simulink model "psbflowsolv"  (Simulink 6.0)
settings: Solver=FixedStepDiscrete  SolverMode=SingleTasking  StartTime=0.0  StopTime=1  FixedStep=0.5  RelTol=1e-3  AbsTol=1e-2
undefined symbols (not defined in the file or in its folder): imag_current_guess, imag_Van_init, Kii, Kir, Pmec, Pref, Qref, R1, r2, real_current_guess, real_Van_init, slip_guess, t_start_current_mot, U, Uref, X1, x2
settings Model: Creator=patrice  LastModifiedBy=batserve  ExtModeTrigMode=oneshot  ExtModeArmWhenConnect=off  ExtModeAutoUpdateStatusClock=off
settings DataIOCC: LimitDataPoints=off  SignalLoggingName=sigsOut
settings OptimizationCC: BooleanDataType=off
settings DebuggingCC: AlgebraicLoopMsg=none  SolverPrmCheckMsg=none  UnconnectedInputMsg=none  UnconnectedOutputMsg=none
settings HardwareCC: TargetUnknown=on
settings RTWCC: TemplateMakefile=grt_unix.tmf

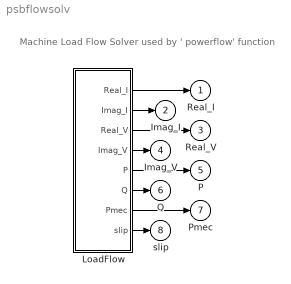
== system psbflowsolv ==
  note: Machine Load Flow Solver
      |  used by ' powerflow' function
  LoadFlow : Subsystem
  Real_I : Outport  InitialOutput=0
  Imag_I : Outport  Port=2  InitialOutput=0
  Real_V : Outport  Port=3  InitialOutput=0
  Imag_V : Outport  Port=4  InitialOutput=0
  P : Outport  Port=5  InitialOutput=0
  Q : Outport  Port=6  InitialOutput=0
  Pmec : Outport  Port=7  InitialOutput=0
  slip : Outport  Port=8  InitialOutput=0
  wires:
  LoadFlow/1(Real_I) -> Real_I/1
  LoadFlow/3(Real_V) -> Real_V/1
  LoadFlow/5(P) -> P/1
  LoadFlow/6(Q) -> Q/1
  LoadFlow/7(Pmec) -> Pmec/1
  LoadFlow/8(slip) -> slip/1
  LoadFlow/4(Imag_V) -> Imag_V/1
  LoadFlow/2(Imag_I) -> Imag_I/1

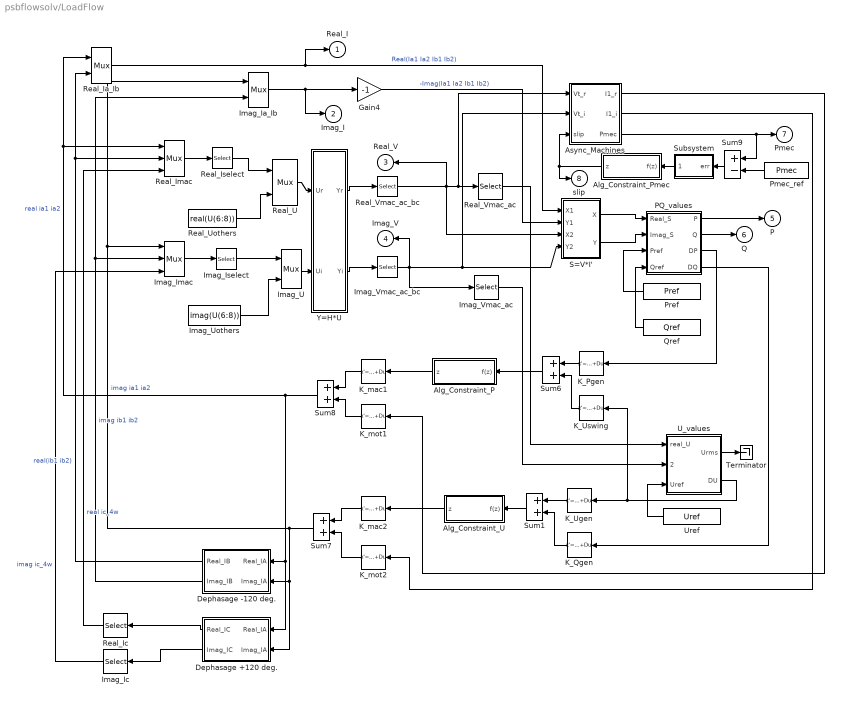
== system psbflowsolv/LoadFlow ==
  Alg_Constraint_P : Subsystem  Orientation=left  mask(Algebraic Constraint){z0=real_current_guess}
      mask prompts: z0 "Initial guess:"
      mask help: Constrains input signal f(z) to zero and outputs an algebraic state z. This block outputs the value necessary to produce a zero at the input. The output must affect the input through some feedback path. Provide an initial guess of the output to improve algebraic loop solver efficiency.
      mask Help:
      | This block outputs the value necessary to produce a zero at the input. The output must affect the input through some feedback path. This allows you to specify algebraic equations for index 1 differential/algebraic systems (DAE's).
      | 
      | By default, the initial guess is zero.  You can improve the efficiency of the algebraic loop solver by providing an initial guess that is close to the solution value.
      mask Display: disp('Solve\nf(z) = 0')
  Alg_Constraint_Pmec : Subsystem  Orientation=left  mask(Algebraic Constraint){z0=slip_guess}
      mask prompts: z0 "Initial guess:"
      mask help: Constrains input signal f(z) to zero and outputs an algebraic state z. This block outputs the value necessary to produce a zero at the input. The output must affect the input through some feedback path. Provide an initial guess of the output to improve algebraic loop solver efficiency.
      mask Help:
      | This block outputs the value necessary to produce a zero at the input. The output must affect the input through some feedback path. This allows you to specify algebraic equations for index 1 differential/algebraic systems (DAE's).
      | 
      | By default, the initial guess is zero.  You can improve the efficiency of the algebraic loop solver by providing an initial guess that is close to the solution value.
      mask Display: disp('Solve\nf(z) = 0')
  Alg_Constraint_U : Subsystem  Orientation=left  mask(Algebraic Constraint){z0=imag_current_guess}
      mask prompts: z0 "Initial guess:"
      mask help: Constrains input signal f(z) to zero and outputs an algebraic state z. This block outputs the value necessary to produce a zero at the input. The output must affect the input through some feedback path. Provide an initial guess of the output to improve algebraic loop solver efficiency.
      mask Help:
      | This block outputs the value necessary to produce a zero at the input. The output must affect the input through some feedback path. This allows you to specify algebraic equations for index 1 differential/algebraic systems (DAE's).
      | 
      | By default, the initial guess is zero.  You can improve the efficiency of the algebraic loop solver by providing an initial guess that is close to the solution value.
      mask Display: disp('Solve\nf(z) = 0')
  Async_Machines : Subsystem
  Dephasage +120 deg. : Subsystem  Orientation=left
  Dephasage -120 deg. : Subsystem  Orientation=left
  Gain4 : Gain  Gain=-1  SaturateOnIntegerOverflow=on
  Imag_Ia_Ib : Mux  Inputs=[2 2]
  Imag_Ic : Selector  Orientation=left  Elements=[1]  InputPortWidth=2
  Imag_Imac : Mux  Inputs=[2 2 1]
  Imag_Iselect : Selector  Elements=[1:5]  InputPortWidth=5
  Imag_U : Mux  Inputs=[5 3]
  Imag_Uothers : Constant  Value=imag(U(6:8))
  Imag_Vmac_ac : Selector  Elements=1:2  InputPortWidth=4
  Imag_Vmac_ac_bc : Selector  Elements=1:4  InputPortWidth=9
  K_Pgen : StateSpace  Orientation=left  A=[]  B=[]  C=[]  D=K  mask(Matrix Gain){@1=[0 0;0 1]}
      mask prompts: @1 "Gain matrix:"
      mask help: Matrix Gain.
      mask init:
      | K=@1;
      mask Help: Multiplies input vector by entered matrix to produce output vector (y=Au).
      mask Display: disp('K')
  K_Qgen : StateSpace  Orientation=left  A=[]  B=[]  C=[]  D=K  mask(Matrix Gain){@1=[0 0;0 1]}
      mask prompts: @1 "Gain matrix:"
      mask help: Matrix Gain.
      mask init:
      | K=@1;
      mask Help: Multiplies input vector by entered matrix to produce output vector (y=Au).
      mask Display: disp('K')
  K_Ugen : StateSpace  Orientation=left  A=[]  B=[]  C=[]  D=K  mask(Matrix Gain){@1=[0 0;0 0]}
      mask prompts: @1 "Gain matrix:"
      mask help: Matrix Gain.
      mask init:
      | K=@1;
      mask Help: Multiplies input vector by entered matrix to produce output vector (y=Au).
      mask Display: disp('K')
  K_Uswing : StateSpace  Orientation=left  A=[]  B=[]  C=[]  D=K  mask(Matrix Gain){@1=[1 0;0 0]}
      mask prompts: @1 "Gain matrix:"
      mask help: Matrix Gain.
      mask init:
      | K=@1;
      mask Help: Multiplies input vector by entered matrix to produce output vector (y=Au).
      mask Display: disp('K')
  K_mac1 : StateSpace  Orientation=left  A=[]  B=[]  C=[]  D=K  mask(Matrix Gain){@1=[1 0;0 1]}
      mask prompts: @1 "Gain matrix:"
      mask help: Matrix Gain.
      mask init:
      | K=@1;
      mask Help: Multiplies input vector by entered matrix to produce output vector (y=Au).
      mask Display: disp('K')
  K_mac2 : StateSpace  Orientation=left  A=[]  B=[]  C=[]  D=K  mask(Matrix Gain){@1=[1 0;0 1]}
      mask prompts: @1 "Gain matrix:"
      mask help: Matrix Gain.
      mask init:
      | K=@1;
      mask Help: Multiplies input vector by entered matrix to produce output vector (y=Au).
      mask Display: disp('K')
  K_mot1 : StateSpace  Orientation=left  A=[]  B=[]  C=[]  D=K  mask(Matrix Gain){@1=[0 0;0 0]}
      mask prompts: @1 "Gain matrix:"
      mask help: Matrix Gain.
      mask init:
      | K=@1;
      mask Help: Multiplies input vector by entered matrix to produce output vector (y=Au).
      mask Display: disp('K')
  K_mot2 : StateSpace  Orientation=left  A=[]  B=[]  C=[]  D=K  mask(Matrix Gain){@1=[0 0;0 0]}
      mask prompts: @1 "Gain matrix:"
      mask help: Matrix Gain.
      mask init:
      | K=@1;
      mask Help: Multiplies input vector by entered matrix to produce output vector (y=Au).
      mask Display: disp('K')
  PQ_values : Subsystem
  Pmec_ref : Constant  Orientation=left  Value=Pmec
  Pref : Constant  Orientation=left  Value=Pref
  Qref : Constant  Orientation=left  Value=Qref
  Real_Ia_Ib : Mux  Inputs=[2 2]
  Real_Ic : Selector  Orientation=left  Elements=[1]  InputPortWidth=2
  Real_Imac : Mux  Inputs=[2 2 1]
  Real_Iselect : Selector  Elements=[1:5]  InputPortWidth=5
  Real_U : Mux  Inputs=[5 3]
  Real_Uothers : Constant  Value=real(U(6:8))
  Real_Vmac_ac : Selector  Elements=1:2  InputPortWidth=4
  Real_Vmac_ac_bc : Selector  Elements=1:4  InputPortWidth=9
  S=V*I' : Subsystem
      mask Display: disp('Z1.*Z2')
  Subsystem : Subsystem  Orientation=left
  Sum{1,6..8} (4 alike) : Sum  Orientation=left  SaturateOnIntegerOverflow=on  InputSameDT=on
  Sum9 : Sum  Orientation=left  Inputs=+-  SaturateOnIntegerOverflow=on  InputSameDT=on
  Terminator : Terminator
  U_values : Subsystem
  Uref : Constant  Orientation=left  Value=Uref
  Y=H*U : Subsystem
      mask Display: disp('Y=H*U')
  Real_I : Outport  InitialOutput=0
  Imag_I : Outport  Port=2  InitialOutput=0
  Real_V : Outport  Orientation=left  Port=3  InitialOutput=0
  Imag_V : Outport  Orientation=left  Port=4  InitialOutput=0
  P : Outport  Port=5  InitialOutput=0
  Q : Outport  Port=6  InitialOutput=0
  Pmec : Outport  Port=7  InitialOutput=0
  slip : Outport  Port=8  InitialOutput=0
  wires:
  Subsystem/1(Psolv) -> Alg_Constraint_Pmec/1(f(z))
  Sum9/1 -> Subsystem/1(err)
  Pmec_ref/1 -> Sum9/2
  Async_Machines/3(Pmec) -> Sum9/1, Pmec/1
  K_mot2/1 -> Sum7/2
  Real_Vmac_ac_bc/1 -> Async_Machines/1(Vt_r), Real_V/1, S=V*I'/3(X2), Real_Vmac_ac/1
  Sum8/1 -> Dephasage -120 deg./1(Real_IA), Dephasage +120 deg./1(Real_IA), Real_Imac/1, Real_Ia_Ib/1  "real ia1 ia2"
  Sum6/1 -> Alg_Constraint_P/1(f(z))
  K_Uswing/1 -> Sum6/2
  K_Pgen/1 -> Sum6/1
  Imag_Vmac_ac_bc/1 -> Async_Machines/2(Vt_i), S=V*I'/4(Y2), Imag_V/1, Imag_Vmac_ac/1
  Real_U/1 -> Y=H*U/1(Ur)
  Y=H*U/2(Yi) -> Imag_Vmac_ac_bc/1
  Y=H*U/1(Yr) -> Real_Vmac_ac_bc/1
  Imag_U/1 -> Y=H*U/2(Ui)
  Gain4/1 -> S=V*I'/2(Y1)  "-Imag(Ia1 Ia2 Ib1 Ib2)"
  U_values/2(DU) -> K_Uswing/1, K_Ugen/1
  PQ_values/2(Q) -> Q/1
  S=V*I'/2(Y) -> PQ_values/2(Imag_S)
  PQ_values/1(P) -> P/1
  Pref/1 -> PQ_values/3(Pref)
  S=V*I'/1(X) -> PQ_values/1(Real_S)
  Imag_Vmac_ac/1 -> U_values/2(imag_U)
  Real_Vmac_ac/1 -> U_values/1(real_U)
  Uref/1 -> U_values/3(Uref)
  PQ_values/3(DP) -> K_Pgen/1
  Imag_Uothers/1 -> Imag_U/2
  Real_Uothers/1 -> Real_U/2
  Alg_Constraint_U/1(z) -> K_mac2/1
  K_mac2/1 -> Sum7/1
  Async_Machines/2(I1_i) -> K_mot2/1
  Dephasage -120 deg./1("Real_IB ") -> Real_Imac/2, Real_Ia_Ib/2  "real(ib1 ib2)"
  Dephasage -120 deg./2("Imag_IB ") -> Imag_Imac/2, Imag_Ia_Ib/2  "imag ib1 ib2"
  Sum7/1 -> Dephasage -120 deg./2(Imag_IA), Dephasage +120 deg./2(Imag_IA), Imag_Imac/1, Imag_Ia_Ib/1  "imag ia1 ia2"
  Alg_Constraint_P/1(z) -> K_mac1/1
  K_mac1/1 -> Sum8/1
  Async_Machines/1(I1_r) -> K_mot1/1
  K_mot1/1 -> Sum8/2
  Alg_Constraint_Pmec/1(z) -> Async_Machines/3(slip), slip/1
  Sum1/1 -> Alg_Constraint_U/1(f(z))
  K_Ugen/1 -> Sum1/1
  K_Qgen/1 -> Sum1/2
  Qref/1 -> PQ_values/4(Qref)
  PQ_values/4(DQ) -> K_Qgen/1
  Dephasage +120 deg./1("Real_IC ") -> Real_Ic/1
  Dephasage +120 deg./2("Imag_IC ") -> Imag_Ic/1
  Real_Ic/1 -> Real_Imac/3  "real ic_4w"
  Imag_Ic/1 -> Imag_Imac/3  "imag ic_4w"
  Real_Ia_Ib/1 -> S=V*I'/1(X1), Real_I/1  "Real(Ia1 Ia2 Ib1 Ib2)"
  Imag_Ia_Ib/1 -> Gain4/1, Imag_I/1
  U_values/1(Urms) -> Terminator/1
  Real_Imac/1 -> Real_Iselect/1
  Real_Iselect/1 -> Real_U/1
  Imag_Imac/1 -> Imag_Iselect/1
  Imag_Iselect/1 -> Imag_U/1

== system psbflowsolv/LoadFlow/Alg_Constraint_P ==
  f(z) : Inport  Port=1  LatchInput=off
  Initial Guess : InitialCondition  Value=z0
  Sum : Sum  SaturateOnIntegerOverflow=on  InputSameDT=on
  z : Outport  InitialOutput=0
  wires:
  Sum/1 -> Initial Guess/1
  Initial Guess/1 -> Sum/2, z/1
  f(z)/1 -> Sum/1

== system psbflowsolv/LoadFlow/Alg_Constraint_Pmec ==
  f(z) : Inport  Port=1  LatchInput=off
  Initial Guess : InitialCondition  Value=z0
  Sum : Sum  SaturateOnIntegerOverflow=on  InputSameDT=on
  z : Outport  InitialOutput=0
  wires:
  f(z)/1 -> Sum/1
  Initial Guess/1 -> z/1, Sum/2
  Sum/1 -> Initial Guess/1

== system psbflowsolv/LoadFlow/Alg_Constraint_U ==
  f(z) : Inport  Port=1  LatchInput=off
  Initial Guess : InitialCondition  Value=z0
  Sum : Sum  SaturateOnIntegerOverflow=on  InputSameDT=on
  z : Outport  InitialOutput=0
  wires:
  Sum/1 -> Initial Guess/1
  Initial Guess/1 -> Sum/2, z/1
  f(z)/1 -> Sum/1

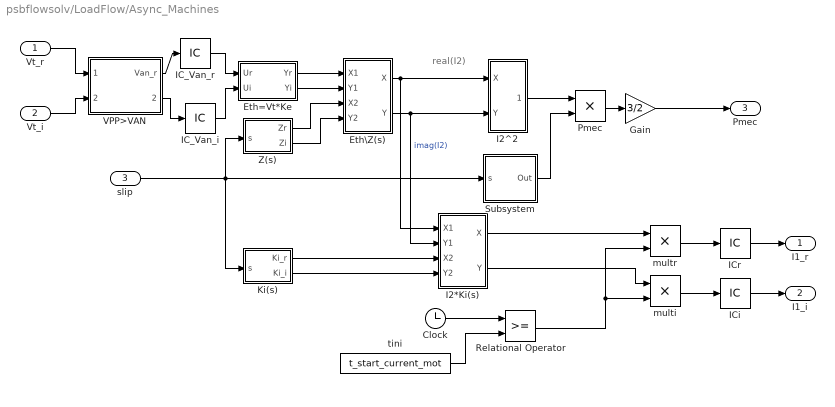
== system psbflowsolv/LoadFlow/Async_Machines ==
  note: real(I2)
  Vt_r : Inport  Port=1  LatchInput=off
  Vt_i : Inport  Port=2  LatchInput=off
  slip : Inport  Port=3  LatchInput=off
  Clock : Clock
      settings: Decimation=10
  Eth=Vt*Ke : Subsystem
      mask Display: disp('Y=H*U')
  Eth\Z(s) : Subsystem
      mask Display: disp('Z1./Z2')
  Gain : Gain  Gain=3/2  SaturateOnIntegerOverflow=on
  I2*Ki(s) : Subsystem
      mask Display: disp('Z1.*Z2')
  I2^2 : Subsystem
  IC_Van_i : InitialCondition  Value=imag_Van_init
  IC_Van_r : InitialCondition  Value=real_Van_init
  ICi : InitialCondition  Value=0
  ICr : InitialCondition  Value=0
  Ki(s) : Subsystem
  "Pmec " : Product  SaturateOnIntegerOverflow=on  InputSameDT=on
  Relational Operator : RelationalOperator  InputSameDT=on
  Subsystem : Subsystem
      mask Display: disp('r2(1-s)/s')
  VPP>VAN : Subsystem
  Z(s) : Subsystem
  "multi " : Product  SaturateOnIntegerOverflow=on  InputSameDT=on
  multr : Product  SaturateOnIntegerOverflow=on  InputSameDT=on
  tini : Constant  Value=t_start_current_mot
  I1_r : Outport  InitialOutput=0
  I1_i : Outport  Port=2  InitialOutput=0
  Pmec : Outport  Port=3  InitialOutput=0
  wires:
  IC_Van_i/1 -> Eth=Vt*Ke/2(Ui)
  VPP>VAN/2(Van_r1) -> IC_Van_i/1
  VPP>VAN/1(Van_r) -> IC_Van_r/1
  IC_Van_r/1 -> Eth=Vt*Ke/1(Ur)
  Relational Operator/1 -> multr/2, "multi "/2
  I2*Ki(s)/2(Y) -> "multi "/1
  I2*Ki(s)/1(X) -> multr/1
  tini/1 -> Relational Operator/2
  Clock/1 -> Relational Operator/1
  Eth\Z(s)/2(Y) -> I2*Ki(s)/2(Y1), I2^2/2(Y)  "imag(I2)"
  Eth\Z(s)/1(X) -> I2*Ki(s)/1(X1), I2^2/1(X)
  Ki(s)/2(Ki_i) -> I2*Ki(s)/4(Y2)
  Ki(s)/1(Ki_r) -> I2*Ki(s)/3(X2)
  Gain/1 -> Pmec/1
  "Pmec "/1 -> Gain/1
  Z(s)/1(Zr) -> Eth\Z(s)/3(X2)
  Z(s)/2(Zi) -> Eth\Z(s)/4(Y2)
  slip/1 -> Ki(s)/1(s), Subsystem/1(s), Z(s)/1(s)
  Subsystem/1(Out) -> "Pmec "/2
  Eth=Vt*Ke/1(Yr) -> Eth\Z(s)/1(X1)
  Eth=Vt*Ke/2(Yi) -> Eth\Z(s)/2(Y1)
  I2^2/1(|Z|^2) -> "Pmec "/1
  multr/1 -> ICr/1
  ICr/1 -> I1_r/1
  "multi "/1 -> ICi/1
  ICi/1 -> I1_i/1
  Vt_r/1 -> VPP>VAN/1(Vac_bc_r)
  Vt_i/1 -> VPP>VAN/2(Vac_bc_i)

== system psbflowsolv/LoadFlow/Dephasage +120 deg. ==
  Real_IA : Inport  Orientation=left  Port=1  LatchInput=off
  Imag_IA : Inport  Orientation=left  Port=2  LatchInput=off
  Mult. complex : Subsystem  Orientation=left
      mask Display: disp('Z1.*Z2')
  imagl(a) : Constant  Orientation=left  Value=sqrt(3)/2
  real(a) : Constant  Orientation=left  Value=-0.5
  "Real_IC " : Outport  Orientation=left  InitialOutput=0
  "Imag_IC " : Outport  Orientation=left  Port=2  InitialOutput=0
  wires:
  Mult. complex/2(Y) -> "Imag_IC "/1
  Mult. complex/1(X) -> "Real_IC "/1
  Real_IA/1 -> Mult. complex/1(X1)
  Imag_IA/1 -> Mult. complex/2(Y1)
  real(a)/1 -> Mult. complex/3(X2)
  imagl(a)/1 -> Mult. complex/4(Y2)

== system psbflowsolv/LoadFlow/Dephasage -120 deg. ==
  Real_IA : Inport  Orientation=left  Port=1  LatchInput=off
  Imag_IA : Inport  Orientation=left  Port=2  LatchInput=off
  Mult. complex : Subsystem  Orientation=left
      mask Display: disp('Z1.*Z2')
  imagl(a^2) : Constant  Orientation=left  Value=-sqrt(3)/2
  real(a^2) : Constant  Orientation=left  Value=-0.5
  "Real_IB " : Outport  Orientation=left  InitialOutput=0
  "Imag_IB " : Outport  Orientation=left  Port=2  InitialOutput=0
  wires:
  imagl(a^2)/1 -> Mult. complex/4(Y2)
  real(a^2)/1 -> Mult. complex/3(X2)
  Imag_IA/1 -> Mult. complex/2(Y1)
  Real_IA/1 -> Mult. complex/1(X1)
  Mult. complex/1(X) -> "Real_IB "/1
  Mult. complex/2(Y) -> "Imag_IB "/1

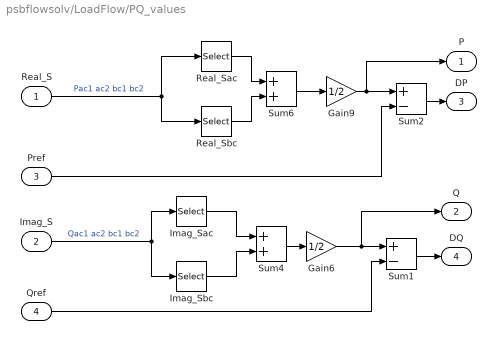
== system psbflowsolv/LoadFlow/PQ_values ==
  Real_S : Inport  Port=1  LatchInput=off
  Imag_S : Inport  Port=2  LatchInput=off
  Pref : Inport  Port=3  LatchInput=off
  Qref : Inport  Port=4  LatchInput=off
  Gain6 : Gain  Gain=1/2  SaturateOnIntegerOverflow=on
  Gain9 : Gain  Gain=1/2  SaturateOnIntegerOverflow=on
  Imag_Sac : Selector  Elements=1:2  InputPortWidth=4
  Imag_Sbc : Selector  Elements=3:4  InputPortWidth=4
  Real_Sac : Selector  Elements=1:2  InputPortWidth=4
  Real_Sbc : Selector  Elements=3:4  InputPortWidth=4
  Sum1 : Sum  Inputs=+-  SaturateOnIntegerOverflow=on  InputSameDT=on
  Sum2 : Sum  Inputs=+-  SaturateOnIntegerOverflow=on  InputSameDT=on
  Sum4 : Sum  SaturateOnIntegerOverflow=on  InputSameDT=on
  Sum6 : Sum  SaturateOnIntegerOverflow=on  InputSameDT=on
  P : Outport  InitialOutput=0
  Q : Outport  Port=2  InitialOutput=0
  DP : Outport  Port=3  InitialOutput=0
  DQ : Outport  Port=4  InitialOutput=0
  wires:
  Imag_S/1 -> Imag_Sac/1, Imag_Sbc/1  "Qac1 ac2 bc1 bc2"
  Sum4/1 -> Gain6/1
  Imag_Sbc/1 -> Sum4/2
  Imag_Sac/1 -> Sum4/1
  Gain9/1 -> P/1, Sum2/1
  Sum2/1 -> DP/1
  Pref/1 -> Sum2/2
  Sum6/1 -> Gain9/1
  Real_Sbc/1 -> Sum6/2
  Real_Sac/1 -> Sum6/1
  Real_S/1 -> Real_Sbc/1, Real_Sac/1  "Pac1 ac2 bc1 bc2"
  Gain6/1 -> Sum1/1, Q/1
  Sum1/1 -> DQ/1
  Qref/1 -> Sum1/2

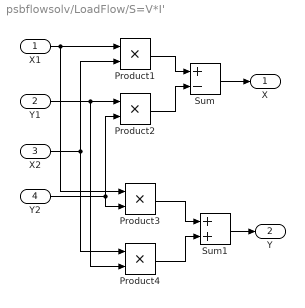
== system psbflowsolv/LoadFlow/S=V*I' ==
  X1 : Inport  Port=1  LatchInput=off
  Y1 : Inport  Port=2  LatchInput=off
  X2 : Inport  Port=3  LatchInput=off
  Y2 : Inport  Port=4  LatchInput=off
  Product{1..4} (4 alike) : Product  SaturateOnIntegerOverflow=on  InputSameDT=on
  Sum : Sum  Inputs=+-  SaturateOnIntegerOverflow=on  InputSameDT=on
  Sum1 : Sum  SaturateOnIntegerOverflow=on  InputSameDT=on
  X : Outport  InitialOutput=0
  Y : Outport  Port=2  InitialOutput=0
  wires:
  Y1/1 -> Product4/2, Product2/1
  X2/1 -> Product4/1, Product1/2
  Y2/1 -> Product3/2, Product2/2
  X1/1 -> Product3/1, Product1/1
  Product3/1 -> Sum1/1
  Product4/1 -> Sum1/2
  Sum1/1 -> Y/1
  Product2/1 -> Sum/2
  Product1/1 -> Sum/1
  Sum/1 -> X/1

== system psbflowsolv/LoadFlow/Subsystem ==
  err : Inport  Port=1  LatchInput=off
  Clock : Clock
      settings: Decimation=10
  Relational Operator : RelationalOperator  InputSameDT=on
  "multi " : Product  SaturateOnIntegerOverflow=on  InputSameDT=on
  tini : Constant  Value=t_start_current_mot
  Psolv : Outport  InitialOutput=0
  wires:
  "multi "/1 -> Psolv/1
  err/1 -> "multi "/1
  tini/1 -> Relational Operator/2
  Clock/1 -> Relational Operator/1
  Relational Operator/1 -> "multi "/2

== system psbflowsolv/LoadFlow/U_values ==
  real_U : Inport  Port=1  LatchInput=off
  imag_U : Inport  Port=2  LatchInput=off
  Uref : Inport  Port=3  LatchInput=off
  Cartesian to Polar2 : Subsystem
      mask Type: Cart2Polar
      mask Description:
      | Transformation from cartesian to polar coordinates.
      | [x, y] -> [r, theta]
      | 
      | r = sqrt(x^2 + y^2);
      | theta = atan(y/x);
      mask Help: Unmask this block for more help.
      mask Display: plot(0,0,100,100,[24,20,15,20,20],[85,95,85,95,20],[80,20,95,85,95,85],[70,20,20,15,20,24],[56,56,55,52,50,46],[20,26,31,35,38,42])
  Sum5 : Sum  Inputs=+-  SaturateOnIntegerOverflow=on  InputSameDT=on
  Vrms : Gain  Gain=1/sqrt(2)  SaturateOnIntegerOverflow=on
  Urms : Outport  InitialOutput=0
  DU : Outport  Port=2  InitialOutput=0
  wires:
  Vrms/1 -> Sum5/1, Urms/1
  real_U/1 -> Cartesian to Polar2/1(x)
  imag_U/1 -> Cartesian to Polar2/2(y)
  Cartesian to Polar2/1(r) -> Vrms/1
  Sum5/1 -> DU/1
  Uref/1 -> Sum5/2

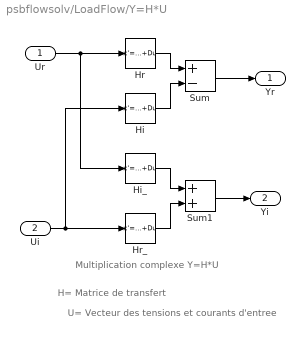
== system psbflowsolv/LoadFlow/Y=H*U ==
  note: Multiplication complexe Y=H*U
  note: H= Matrice de transfert
  note: U= Vecteur des tensions et courants d'entree
  Ur : Inport  Port=1  LatchInput=off
  Ui : Inport  Port=2  LatchInput=off
  Hi : StateSpace  A=[]  B=[]  C=[]  D=K  mask(Matrix Gain){@1=imag(H)}
      mask prompts: @1 "Gain matrix:"
      mask help: Matrix Gain.
      mask init:
      | K=@1;
      mask Help: Multiplies input vector by entered matrix to produce output vector (y=Au).
      mask Display: disp('K')
  Hi_ : StateSpace  A=[]  B=[]  C=[]  D=K  mask(Matrix Gain){@1=imag(H)}
      mask prompts: @1 "Gain matrix:"
      mask help: Matrix Gain.
      mask init:
      | K=@1;
      mask Help: Multiplies input vector by entered matrix to produce output vector (y=Au).
      mask Display: disp('K')
  Hr : StateSpace  A=[]  B=[]  C=[]  D=K  mask(Matrix Gain){@1=real(H)}
      mask prompts: @1 "Gain matrix:"
      mask help: Matrix Gain.
      mask init:
      | K=@1;
      mask Help: Multiplies input vector by entered matrix to produce output vector (y=Au).
      mask Display: disp('K')
  Hr_ : StateSpace  A=[]  B=[]  C=[]  D=K  mask(Matrix Gain){@1=real(H)}
      mask prompts: @1 "Gain matrix:"
      mask help: Matrix Gain.
      mask init:
      | K=@1;
      mask Help: Multiplies input vector by entered matrix to produce output vector (y=Au).
      mask Display: disp('K')
  Sum : Sum  Inputs=+-  SaturateOnIntegerOverflow=on  InputSameDT=on
  Sum1 : Sum  SaturateOnIntegerOverflow=on  InputSameDT=on
  Yr : Outport  InitialOutput=0
  Yi : Outport  Port=2  InitialOutput=0
  wires:
  Hr/1 -> Sum/1
  Hi/1 -> Sum/2
  Sum/1 -> Yr/1
  Ur/1 -> Hr/1, Hi_/1
  Ui/1 -> Hi/1, Hr_/1
  Hi_/1 -> Sum1/1
  Hr_/1 -> Sum1/2
  Sum1/1 -> Yi/1

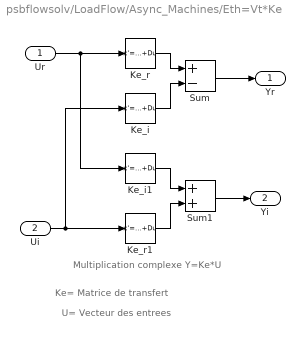
== system psbflowsolv/LoadFlow/Async_Machines/Eth=Vt*Ke ==
  note: Multiplication complexe Y=Ke*U
  note: Ke= Matrice de transfert
  note: U= Vecteur des entrees
  Ur : Inport  Port=1  LatchInput=off
  Ui : Inport  Port=2  LatchInput=off
  Ke_i : StateSpace  A=[]  B=[]  C=[]  D=K  mask(Matrix Gain){@1=imag(Ke)}
      mask prompts: @1 "Gain matrix:"
      mask help: Matrix Gain.
      mask init:
      | K=@1;
      mask Help: Multiplies input vector by entered matrix to produce output vector (y=Au).
      mask Display: disp('K')
  Ke_i1 : StateSpace  A=[]  B=[]  C=[]  D=K  mask(Matrix Gain){@1=imag(Ke)}
      mask prompts: @1 "Gain matrix:"
      mask help: Matrix Gain.
      mask init:
      | K=@1;
      mask Help: Multiplies input vector by entered matrix to produce output vector (y=Au).
      mask Display: disp('K')
  Ke_r : StateSpace  A=[]  B=[]  C=[]  D=K  mask(Matrix Gain){@1=real(Ke)}
      mask prompts: @1 "Gain matrix:"
      mask help: Matrix Gain.
      mask init:
      | K=@1;
      mask Help: Multiplies input vector by entered matrix to produce output vector (y=Au).
      mask Display: disp('K')
  Ke_r1 : StateSpace  A=[]  B=[]  C=[]  D=K  mask(Matrix Gain){@1=real(Ke)}
      mask prompts: @1 "Gain matrix:"
      mask help: Matrix Gain.
      mask init:
      | K=@1;
      mask Help: Multiplies input vector by entered matrix to produce output vector (y=Au).
      mask Display: disp('K')
  Sum : Sum  Inputs=+-  SaturateOnIntegerOverflow=on  InputSameDT=on
  Sum1 : Sum  SaturateOnIntegerOverflow=on  InputSameDT=on
  Yr : Outport  InitialOutput=0
  Yi : Outport  Port=2  InitialOutput=0
  wires:
  Ke_r/1 -> Sum/1
  Ke_i/1 -> Sum/2
  Sum/1 -> Yr/1
  Ui/1 -> Ke_i/1, Ke_r1/1
  Ke_i1/1 -> Sum1/1
  Ke_r1/1 -> Sum1/2
  Sum1/1 -> Yi/1
  Ur/1 -> Ke_r/1, Ke_i1/1

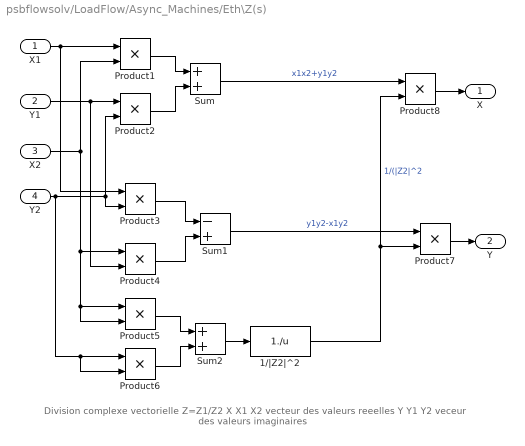
== system psbflowsolv/LoadFlow/Async_Machines/Eth\Z(s) ==
  note: Division complexe vectorielle Z=Z1/Z2
      | X X1 X2 vecteur des valeurs reeelles
      | Y Y1 Y2 veceur des valeurs imaginaires
  X1 : Inport  Port=1  LatchInput=off
  Y1 : Inport  Port=2  LatchInput=off
  X2 : Inport  Port=3  LatchInput=off
  Y2 : Inport  Port=4  LatchInput=off
  1/|Z2|^2 : MATLABFcn  MATLABFcn=1./u
  Product{1..8} (8 alike) : Product  SaturateOnIntegerOverflow=on  InputSameDT=on
  Sum : Sum  SaturateOnIntegerOverflow=on  InputSameDT=on
  Sum1 : Sum  Inputs=-+  SaturateOnIntegerOverflow=on  InputSameDT=on
  Sum2 : Sum  SaturateOnIntegerOverflow=on  InputSameDT=on
  X : Outport  InitialOutput=0
  Y : Outport  Port=2  InitialOutput=0
  wires:
  Product8/1 -> X/1
  Product7/1 -> Y/1
  Sum1/1 -> Product7/1  "y1y2-x1y2"
  1/|Z2|^2/1 -> Product8/2, Product7/2  "1/(|Z2|^2"
  Sum/1 -> Product8/1  "x1x2+y1y2"
  Sum2/1 -> 1/|Z2|^2/1
  Product6/1 -> Sum2/2
  Product5/1 -> Sum2/1
  Y2/1 -> Product6/2, Product6/1, Product3/2, Product2/2
  Y1/1 -> Product4/2, Product2/1
  X2/1 -> Product5/2, Product5/1, Product4/1, Product1/2
  X1/1 -> Product3/1, Product1/1
  Product3/1 -> Sum1/1
  Product4/1 -> Sum1/2
  Product2/1 -> Sum/2
  Product1/1 -> Sum/1

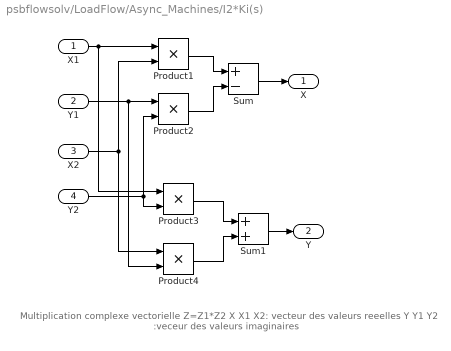
== system psbflowsolv/LoadFlow/Async_Machines/I2*Ki(s) ==
  note: Multiplication  complexe vectorielle Z=Z1*Z2
      | X X1 X2:  vecteur des valeurs reeelles
      | Y Y1 Y2 :veceur des valeurs imaginaires
  X1 : Inport  Port=1  LatchInput=off
  Y1 : Inport  Port=2  LatchInput=off
  X2 : Inport  Port=3  LatchInput=off
  Y2 : Inport  Port=4  LatchInput=off
  Product{1..4} (4 alike) : Product  SaturateOnIntegerOverflow=on  InputSameDT=on
  Sum : Sum  Inputs=+-  SaturateOnIntegerOverflow=on  InputSameDT=on
  Sum1 : Sum  SaturateOnIntegerOverflow=on  InputSameDT=on
  X : Outport  InitialOutput=0
  Y : Outport  Port=2  InitialOutput=0
  wires:
  Y1/1 -> Product4/2, Product2/1
  X2/1 -> Product4/1, Product1/2
  Y2/1 -> Product3/2, Product2/2
  X1/1 -> Product3/1, Product1/1
  Product3/1 -> Sum1/1
  Product4/1 -> Sum1/2
  Sum1/1 -> Y/1
  Product2/1 -> Sum/2
  Product1/1 -> Sum/1
  Sum/1 -> X/1

== system psbflowsolv/LoadFlow/Async_Machines/I2^2 ==
  X : Inport  Port=1  LatchInput=off
  Y : Inport  Port=2  LatchInput=off
  Product5 : Product  SaturateOnIntegerOverflow=on  InputSameDT=on
  Product6 : Product  SaturateOnIntegerOverflow=on  InputSameDT=on
  Sum2 : Sum  SaturateOnIntegerOverflow=on  InputSameDT=on
  |Z|^2 : Outport  InitialOutput=0
  wires:
  Product5/1 -> Sum2/1
  Product6/1 -> Sum2/2
  Sum2/1 -> |Z|^2/1
  X/1 -> Product5/1, Product5/2
  Y/1 -> Product6/1, Product6/2

== system psbflowsolv/LoadFlow/Async_Machines/Ki(s) ==
  s : Inport  Port=1  LatchInput=off
  1/s : MATLABFcn  MATLABFcn=1./u
  Kii : Constant  Value=Kii
  Kii/s : Product  SaturateOnIntegerOverflow=on  InputSameDT=on
  Kir : Constant  Value=Kir
  Ki_r : Outport  InitialOutput=0
  Ki_i : Outport  Port=2  InitialOutput=0
  wires:
  Kii/s/1 -> Ki_i/1
  Kir/1 -> Ki_r/1
  1/s/1 -> Kii/s/1
  Kii/1 -> Kii/s/2
  s/1 -> 1/s/1

== system psbflowsolv/LoadFlow/Async_Machines/Subsystem ==
  s : Inport  Port=1  LatchInput=off
  (1-s) : Sum  Inputs=+-  SaturateOnIntegerOverflow=on  InputSameDT=on
  (1-s)\s : Product  SaturateOnIntegerOverflow=on  InputSameDT=on
  1 : Constant
  1\s : MATLABFcn  MATLABFcn=1./u
  mult : Product  SaturateOnIntegerOverflow=on  InputSameDT=on
  r2 : Constant  Value=r2
  Out : Outport  InitialOutput=0
  wires:
  mult/1 -> Out/1
  1/1 -> (1-s)/1
  (1-s)/1 -> (1-s)\s/1
  1\s/1 -> (1-s)\s/2
  (1-s)\s/1 -> mult/1
  r2/1 -> mult/2
  s/1 -> (1-s)/2, 1\s/1

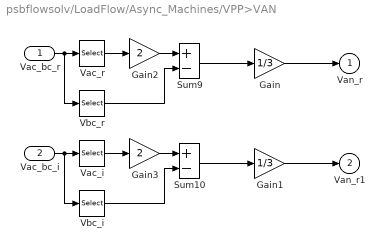
== system psbflowsolv/LoadFlow/Async_Machines/VPP>VAN ==
  Vac_bc_r : Inport  Port=1  LatchInput=off
  Vac_bc_i : Inport  Port=2  LatchInput=off
  Gain : Gain  Gain=1/3  SaturateOnIntegerOverflow=on
  Gain1 : Gain  Gain=1/3  SaturateOnIntegerOverflow=on
  Gain2 : Gain  Gain=2  SaturateOnIntegerOverflow=on
  Gain3 : Gain  Gain=2  SaturateOnIntegerOverflow=on
  Sum10 : Sum  Inputs=+-  SaturateOnIntegerOverflow=on  InputSameDT=on
  Sum9 : Sum  Inputs=+-  SaturateOnIntegerOverflow=on  InputSameDT=on
  Vac_i : Selector  Elements=1:2  InputPortWidth=4
  Vac_r : Selector  Elements=1:2  InputPortWidth=4
  Vbc_i : Selector  Elements=3:4  InputPortWidth=4
  Vbc_r : Selector  Elements=3:4  InputPortWidth=4
  Van_r : Outport  InitialOutput=0
  Van_r1 : Outport  Port=2  InitialOutput=0
  wires:
  Gain/1 -> Van_r/1
  Sum9/1 -> Gain/1
  Gain1/1 -> Van_r1/1
  Sum10/1 -> Gain1/1
  Vbc_i/1 -> Sum10/2
  Vac_bc_i/1 -> Vac_i/1, Vbc_i/1
  Vac_i/1 -> Gain3/1
  Gain3/1 -> Sum10/1
  Vbc_r/1 -> Sum9/2
  Vac_bc_r/1 -> Vbc_r/1, Vac_r/1
  Vac_r/1 -> Gain2/1
  Gain2/1 -> Sum9/1

== system psbflowsolv/LoadFlow/Async_Machines/Z(s) ==
  s : Inport  Port=1  LatchInput=off
  1/s : MATLABFcn  MATLABFcn=1./u
  R1 : Constant  Value=R1
  Sum : Sum  SaturateOnIntegerOverflow=on  InputSameDT=on
  X1+x2 : Constant  Value=X1+x2
  r2 : Constant  Value=r2
  r2/s : Product  SaturateOnIntegerOverflow=on  InputSameDT=on
  Zr : Outport  InitialOutput=0
  Zi : Outport  Port=2  InitialOutput=0
  wires:
  R1/1 -> Sum/1
  Sum/1 -> Zr/1
  s/1 -> 1/s/1
  X1+x2/1 -> Zi/1
  r2/1 -> r2/s/2
  1/s/1 -> r2/s/1
  r2/s/1 -> Sum/2

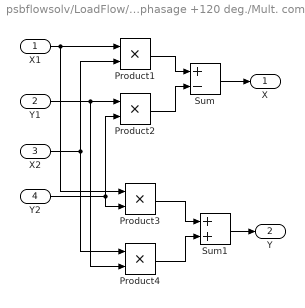
== system psbflowsolv/LoadFlow/Dephasage +120 deg./Mult. complex ==
  X1 : Inport  Port=1  LatchInput=off
  Y1 : Inport  Port=2  LatchInput=off
  X2 : Inport  Port=3  LatchInput=off
  Y2 : Inport  Port=4  LatchInput=off
  Product{1..4} (4 alike) : Product  SaturateOnIntegerOverflow=on  InputSameDT=on
  Sum : Sum  Inputs=+-  SaturateOnIntegerOverflow=on  InputSameDT=on
  Sum1 : Sum  SaturateOnIntegerOverflow=on  InputSameDT=on
  X : Outport  InitialOutput=0
  Y : Outport  Port=2  InitialOutput=0
  wires:
  Y1/1 -> Product4/2, Product2/1
  X2/1 -> Product4/1, Product1/2
  Y2/1 -> Product3/2, Product2/2
  X1/1 -> Product3/1, Product1/1
  Product3/1 -> Sum1/1
  Product4/1 -> Sum1/2
  Sum1/1 -> Y/1
  Product2/1 -> Sum/2
  Product1/1 -> Sum/1
  Sum/1 -> X/1

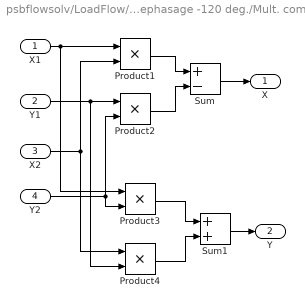
== system psbflowsolv/LoadFlow/Dephasage -120 deg./Mult. complex ==
  X1 : Inport  Port=1  LatchInput=off
  Y1 : Inport  Port=2  LatchInput=off
  X2 : Inport  Port=3  LatchInput=off
  Y2 : Inport  Port=4  LatchInput=off
  Product{1..4} (4 alike) : Product  SaturateOnIntegerOverflow=on  InputSameDT=on
  Sum : Sum  Inputs=+-  SaturateOnIntegerOverflow=on  InputSameDT=on
  Sum1 : Sum  SaturateOnIntegerOverflow=on  InputSameDT=on
  X : Outport  InitialOutput=0
  Y : Outport  Port=2  InitialOutput=0
  wires:
  Sum/1 -> X/1
  Product1/1 -> Sum/1
  Product2/1 -> Sum/2
  Sum1/1 -> Y/1
  Product4/1 -> Sum1/2
  Product3/1 -> Sum1/1
  X1/1 -> Product1/1, Product3/1
  Y2/1 -> Product2/2, Product3/2
  X2/1 -> Product1/2, Product4/1
  Y1/1 -> Product2/1, Product4/2

== system psbflowsolv/LoadFlow/U_values/Cartesian to Polar2 ==
  x : Inport  Port=1  LatchInput=off
  y : Inport  Port=2  LatchInput=off
  Product : Product  SaturateOnIntegerOverflow=on  InputSameDT=on
  Product1 : Product  SaturateOnIntegerOverflow=on  InputSameDT=on
  Sum : Sum  SaturateOnIntegerOverflow=on  InputSameDT=on
  sqrt : MATLABFcn  MATLABFcn=sqrt(u)
  r : Outport  InitialOutput=0
  wires:
  y/1 -> Product/2, Product/1
  x/1 -> Product1/2, Product1/1
  sqrt/1 -> r/1
  Sum/1 -> sqrt/1
  Product/1 -> Sum/2
  Product1/1 -> Sum/1
